simulink model "Black_box_system_2_1_3"  (R2025b)
settings: Solver=VariableStepAuto  StartTime=0.0  StopTime=20  FixedStep=0.001  RelTol=1e-3
undefined symbols (not defined in the file): Beq, degs2rpm, drv, gbox, Jeq, K_W, kd, ki, kp, mld, mot, rdp, Req, sens, tl, u_bar_max
libraries: simulink x1
settings Model: Creator=Enrico  LastModifiedBy=Enrico
settings DataIOCC: ReturnWorkspaceOutputsName=out_black_box

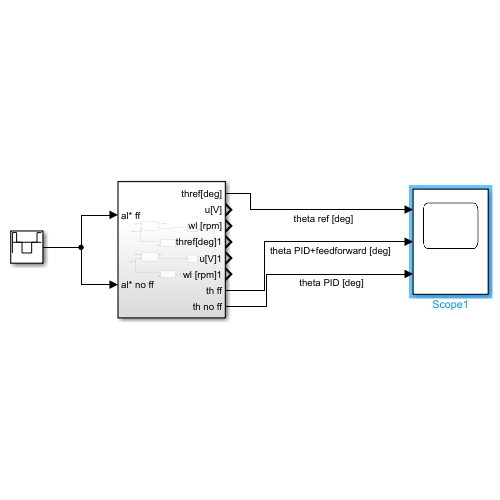
[thumbnail: Simulink's stored preview of the top-level diagram]
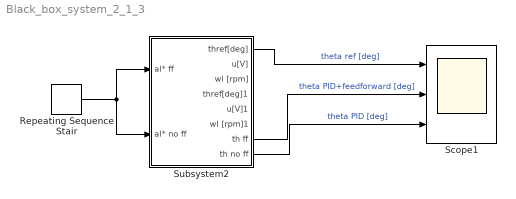
== system Black_box_system_2_1_3 ==
  Repeating Sequence Stair : simulink/Sources/Repeating Sequence Stair  OutValues=[900 0 -900 -900 0 900]  tsamp=0.5  OutMin=[]  OutMax=[]  OutDataTypeStr=double  OutputDataTypeScalingMode=double  OutDataType=fixdt(0,8)  ConRadixGroup=Best Precision: Vector-wise  OutScaling=2^-12
  Scope1 : Scope  NumInputPorts=3
      settings: ActiveDisplayYMinimum=2541.6022792553317  ActiveDisplayYMaximum=2555.3739505789249
  Subsystem2 : Subsystem
  wires:
  Repeating Sequence Stair/1 -> Subsystem2/2(al* no ff), Subsystem2/1(al* ff)
  Subsystem2/1(thref[deg]) -> Scope1/1  "theta ref [deg]"
  Subsystem2/8(th no ff) -> Scope1/3  "theta PID [deg]"
  Subsystem2/7(th ff) -> Scope1/2  "theta PID+feedforward [deg]"

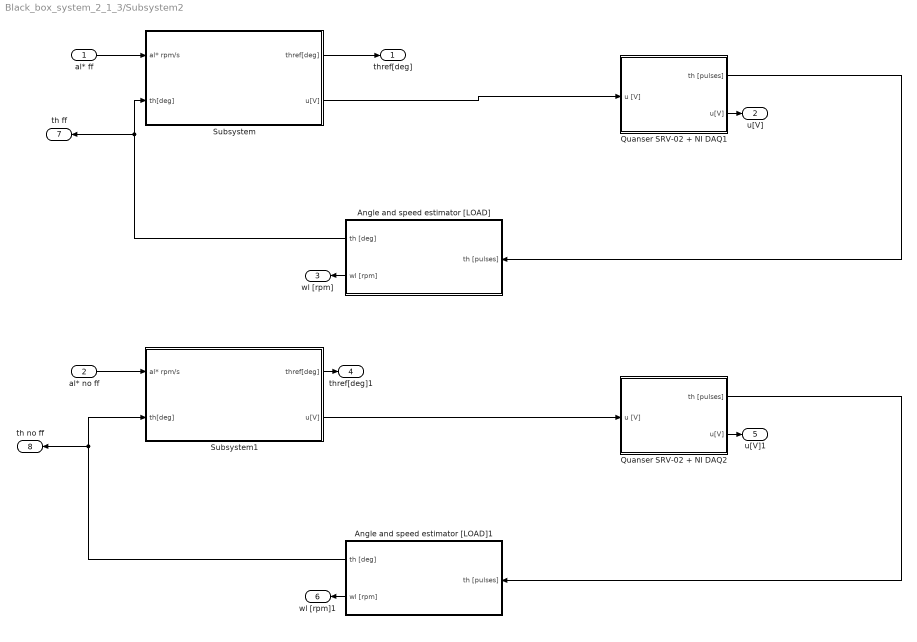
== system Black_box_system_2_1_3/Subsystem2 ==
  al* ff : Inport
  al* no ff : Inport  Port=2
  Angle and speed estimator [LOAD] : Subsystem
  Angle and speed estimator [LOAD]1 : Subsystem
  Quanser SRV-02 + NI DAQ1 : Subsystem  mask(Quanser SRV-02 (with inertial load) + NI DAQ){Ts=0.001, fricType=Karnopp}
      mask prompts: Ts "NI DAQ Sample Time:"; fricType "Friction model"
      mask help: Quanser SRV-02 (with inertial load) + NI DAQ model.
      mask init:
      | %%  Sensors data
      | 
      | %   shunt resistor
      | sens.curr.Rs = 0.5;                         %   resistance [Ohm]   
      | sens.curr.uRs_std = 0.01;                   %   voltage noise standard dev [V]                           
      | sens.curr.uRs_var = sens.curr.uRs_std^2;	%   voltage noise variance [V^2]
      | 
      | %   Hewlett-Packard HEDS-5540#A06 optical encoder
      | sens.enc.ppr = 500*4;                       %   pulses per rotation
      | sens.enc.pulse2deg = 360/sens.enc.ppr;      %   [pulses] -> [deg]
      | sens.enc.pulse2rad = 2*pi/sens.enc.ppr;     %   [pulses] -> [rad]
      | sens.enc.deg2pulse = sens.enc.ppr/360;      %   [deg] -> [pulses]
      | sens.enc.rad2pulse = sens.enc.ppr/2/pi;     %   [rad] -> [pulses]
      | 
      | 
      | %%  Data acquisition board (daq) data
      | 
      | %   NI PCI-6221 DAC data
      | daq.dac.bits = 16;                                  %   resolution (bits)
      | daq.dac.fs   = 10;                                  %   full scale 
      | daq.dac.q    = 2*daq.dac.fs/(2^daq.dac.bits-1);     %	quantization
      | 
      | %   NI PCI-6221 ADC data
      | daq.adc.bits = 16;                                  %   resolution (bits)
      | daq.adc.fs   = 10;                                  %   full scale (as set in SLDRT Analog Input block)
      | daq.adc.q    = 2*daq.adc.fs/(2^daq.adc.bits-1);     %   quantization
      mask Help:
      | Riccardo Antonello (antonello@dei.unipd.it)
      | 
      | April 24, 2020
      | 
      | Dept. of Information Engineering, University of Padova
      mask TypeOptions fricType: Coulomb + viscous | Karnopp
  Quanser SRV-02 + NI DAQ2 : Subsystem  mask(Quanser SRV-02 (with inertial load) + NI DAQ){Ts=0.001, fricType=Karnopp}
      mask prompts: Ts "NI DAQ Sample Time:"; fricType "Friction model"
      mask help: Quanser SRV-02 (with inertial load) + NI DAQ model.
      mask init: same as Black_box_system_2_1_3/Subsystem2/Quanser SRV-02 + NI DAQ1
      mask Help:
      | Riccardo Antonello (antonello@dei.unipd.it)
      | 
      | April 24, 2020
      | 
      | Dept. of Information Engineering, University of Padova
      mask TypeOptions fricType: Coulomb + viscous | Karnopp
  Subsystem : Subsystem
  Subsystem1 : Subsystem
  thref[deg] : Outport
  u[V] : Outport  Port=2
  wl [rpm] : Outport  Port=3
  thref[deg]1 : Outport  Port=4
  u[V]1 : Outport  Port=5
  wl [rpm]1 : Outport  Port=6
  th ff : Outport  Port=7
  th no ff : Outport  Port=8
  wires:
  Subsystem/2(u[V]) -> Quanser SRV-02 + NI DAQ1/1(u [V])
  al* no ff/1 -> Subsystem1/1(al* rpm/s)
  Quanser SRV-02 + NI DAQ1/1(th [pulses]) -> Angle and speed estimator [LOAD]/1(th [pulses])
  Angle and speed estimator [LOAD]1/1(th [deg]) -> Subsystem1/2(th[deg]), th no ff/1
  Subsystem1/2(u[V]) -> Quanser SRV-02 + NI DAQ2/1(u [V])
  Quanser SRV-02 + NI DAQ2/2(u[V]) -> u[V]1/1
  Quanser SRV-02 + NI DAQ2/1(th [pulses]) -> Angle and speed estimator [LOAD]1/1(th [pulses])
  Angle and speed estimator [LOAD]/1(th [deg]) -> th ff/1, Subsystem/2(th[deg])
  Subsystem/1(thref[deg]) -> thref[deg]/1
  al* ff/1 -> Subsystem/1(al* rpm/s)
  Angle and speed estimator [LOAD]1/2(wl [rpm]) -> wl [rpm]1/1
  Angle and speed estimator [LOAD]/2(wl [rpm]) -> wl [rpm]/1
  Subsystem1/1(thref[deg]) -> thref[deg]1/1
  Quanser SRV-02 + NI DAQ1/2(u[V]) -> u[V]/1

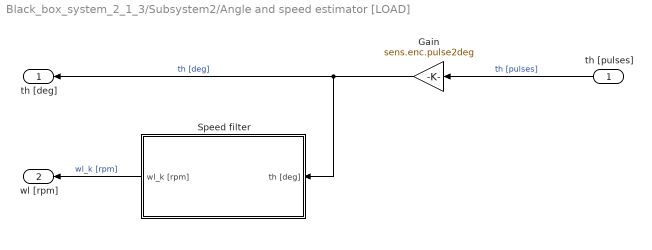
== system Black_box_system_2_1_3/Subsystem2/Angle and speed estimator [LOAD] ==
  th [pulses] : Inport
  Gain : Gain  Gain=sens.enc.pulse2deg
  Speed filter : Subsystem
  th [deg] : Outport
  wl [rpm] : Outport  Port=2
  wires:
  Speed filter/1(wl_k [rpm]) -> wl [rpm]/1  "wl_k [rpm]"
  th [pulses]/1 -> Gain/1  "th [pulses]"
  Gain/1 -> Speed filter/1(th [deg]), th [deg]/1  "th [deg]"

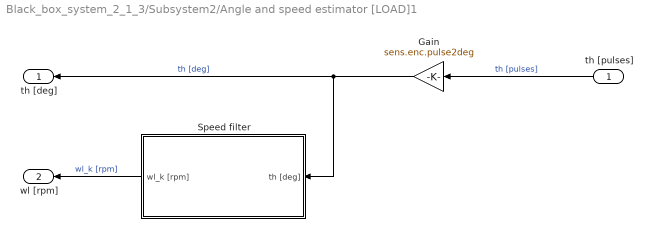
== system Black_box_system_2_1_3/Subsystem2/Angle and speed estimator [LOAD]1 ==
  th [pulses] : Inport
  Gain : Gain  Gain=sens.enc.pulse2deg
  Speed filter : Subsystem
  th [deg] : Outport
  wl [rpm] : Outport  Port=2
  wires:
  Speed filter/1(wl_k [rpm]) -> wl [rpm]/1  "wl_k [rpm]"
  th [pulses]/1 -> Gain/1  "th [pulses]"
  Gain/1 -> Speed filter/1(th [deg]), th [deg]/1  "th [deg]"

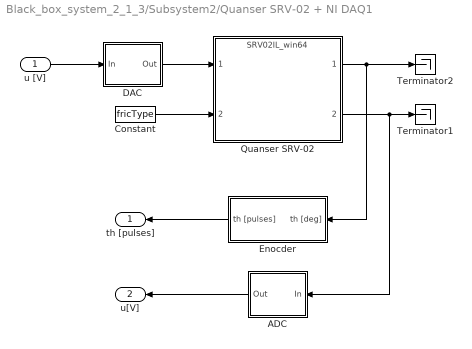
== system Black_box_system_2_1_3/Subsystem2/Quanser SRV-02 + NI DAQ1 ==
  u [V] : Inport
  ADC : Subsystem
  Constant : Constant  Value=fricType
  DAC : Subsystem
  Enocder : Subsystem
  Quanser SRV-02 : ModelReference  ModelNameDialog=SRV02IL_win64.slxp  ModelReferenceVersion=1.44  CopyOfModelProtected=on
  Terminator1 : Terminator
  Terminator2 : Terminator
  th [pulses] : Outport
  u[V] : Outport  Port=2
  wires:
  Enocder/1(th [pulses]) -> th [pulses]/1
  ADC/1(Out) -> u[V]/1
  DAC/1(Out) -> Quanser SRV-02/1
  Quanser SRV-02/2 -> ADC/1(In), Terminator1/1
  u [V]/1 -> DAC/1(In)
  Quanser SRV-02/1 -> Enocder/1(th [deg]), Terminator2/1
  Constant/1 -> Quanser SRV-02/2

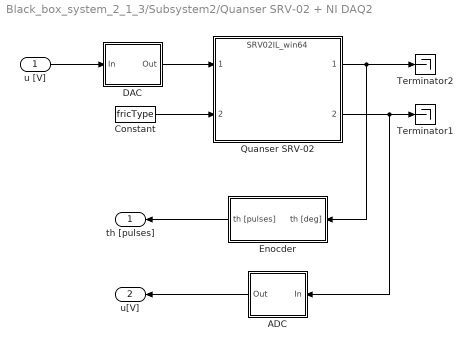
== system Black_box_system_2_1_3/Subsystem2/Quanser SRV-02 + NI DAQ2 ==
  u [V] : Inport
  ADC : Subsystem
  Constant : Constant  Value=fricType
  DAC : Subsystem
  Enocder : Subsystem
  Quanser SRV-02 : ModelReference  ModelNameDialog=SRV02IL_win64.slxp  ModelReferenceVersion=1.44  CopyOfModelProtected=on
  Terminator1 : Terminator
  Terminator2 : Terminator
  th [pulses] : Outport
  u[V] : Outport  Port=2
  wires:
  Enocder/1(th [pulses]) -> th [pulses]/1
  ADC/1(Out) -> u[V]/1
  DAC/1(Out) -> Quanser SRV-02/1
  Quanser SRV-02/2 -> ADC/1(In), Terminator1/1
  u [V]/1 -> DAC/1(In)
  Quanser SRV-02/1 -> Enocder/1(th [deg]), Terminator2/1
  Constant/1 -> Quanser SRV-02/2

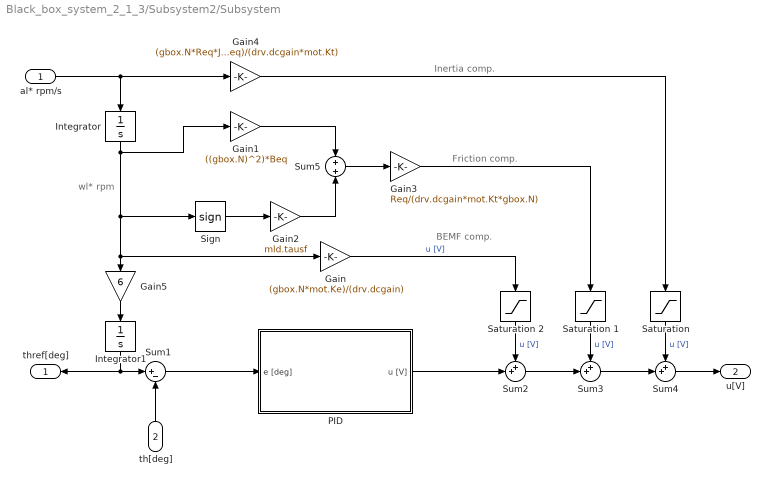
== system Black_box_system_2_1_3/Subsystem2/Subsystem ==
  note: rpm
  note: Inertia comp.
  note: Friction comp.
  note: BEMF comp.
  note: wl*
  al* rpm/s : Inport
  th[deg] : Inport  Port=2
  Gain : Gain  Gain=(gbox.N*mot.Ke)/(drv.dcgain)
  Gain1 : Gain  Gain=((gbox.N)^2)*Beq
  Gain2 : Gain  Gain=mld.tausf
  Gain3 : Gain  Gain=Req/(drv.dcgain*mot.Kt*gbox.N)
  Gain4 : Gain  Gain=(gbox.N*Req*Jeq)/(drv.dcgain*mot.Kt)
  Gain5 : Gain  Gain=6
  Integrator : Integrator
  Integrator1 : Integrator
  PID : Subsystem
  "Saturation " : Saturate  UpperLimit=u_bar_max  LowerLimit=-u_bar_max
  Saturation 1 : Saturate  UpperLimit=u_bar_max  LowerLimit=-u_bar_max
  Saturation 2 : Saturate  UpperLimit=u_bar_max  LowerLimit=-u_bar_max
  Sign : Signum
  Sum1 : Sum  Inputs=|+-
  Sum2 : Sum  Inputs=++|
  Sum3 : Sum  Inputs=++|
  Sum4 : Sum  Inputs=++|
  Sum5 : Sum  Inputs=+|+
  thref[deg] : Outport
  u[V] : Outport  Port=2
  wires:
  Sum3/1 -> Sum4/2
  Gain2/1 -> Sum5/2
  Integrator/1 -> Sign/1, Gain5/1, Gain/1, Gain1/1
  Sum2/1 -> Sum3/2
  Sum4/1 -> u[V]/1
  Integrator1/1 -> thref[deg]/1, Sum1/1
  Saturation 1/1 -> Sum3/1  "u [V]"
  PID/1(u [V]) -> Sum2/2
  Sum5/1 -> Gain3/1
  Gain1/1 -> Sum5/1
  Gain5/1 -> Integrator1/1
  Sign/1 -> Gain2/1
  Saturation 2/1 -> Sum2/1  "u [V]"
  Sum1/1 -> PID/1(e [deg])
  "Saturation "/1 -> Sum4/1  "u [V]"
  al* rpm/s/1 -> Gain4/1, Integrator/1
  th[deg]/1 -> Sum1/2
  Gain4/1 -> "Saturation "/1
  Gain3/1 -> Saturation 1/1
  Gain/1 -> Saturation 2/1  "u [V]"

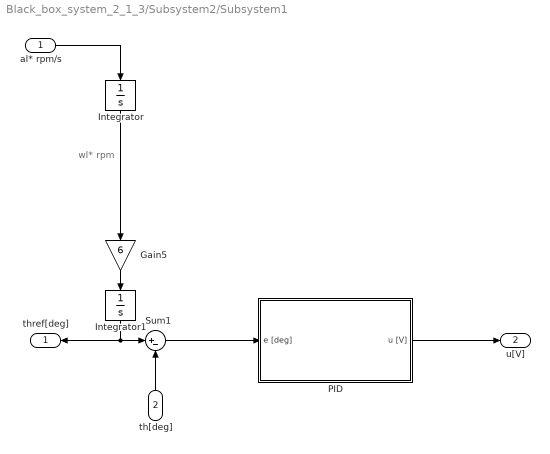
== system Black_box_system_2_1_3/Subsystem2/Subsystem1 ==
  note: rpm
  note: wl*
  al* rpm/s : Inport
  th[deg] : Inport  Port=2
  Gain5 : Gain  Gain=6
  Integrator : Integrator
  Integrator1 : Integrator
  PID : Subsystem
  Sum1 : Sum  Inputs=|+-
  thref[deg] : Outport
  u[V] : Outport  Port=2
  wires:
  Integrator/1 -> Gain5/1
  Integrator1/1 -> thref[deg]/1, Sum1/1
  Gain5/1 -> Integrator1/1
  Sum1/1 -> PID/1(e [deg])
  al* rpm/s/1 -> Integrator/1
  th[deg]/1 -> Sum1/2
  PID/1(u [V]) -> u[V]/1

== system Black_box_system_2_1_3/Subsystem2/Angle and speed estimator [LOAD]/Speed filter ==
  th [deg] : Inport
  Real Derivative : TransferFcn  Numerator=[rdp.wci^2 0]  Denominator=[1 2*rdp.di*rdp.wci rdp.wci^2]
  degs2rpm : Gain  Gain=degs2rpm
  wl_k [rpm] : Outport
  wires:
  th [deg]/1 -> Real Derivative/1
  degs2rpm/1 -> wl_k [rpm]/1  "wl-meas"
  Real Derivative/1 -> degs2rpm/1

== system Black_box_system_2_1_3/Subsystem2/Angle and speed estimator [LOAD]1/Speed filter ==
  th [deg] : Inport
  Real Derivative : TransferFcn  Numerator=[rdp.wci^2 0]  Denominator=[1 2*rdp.di*rdp.wci rdp.wci^2]
  degs2rpm : Gain  Gain=degs2rpm
  wl_k [rpm] : Outport
  wires:
  th [deg]/1 -> Real Derivative/1
  degs2rpm/1 -> wl_k [rpm]/1  "wl-meas"
  Real Derivative/1 -> degs2rpm/1

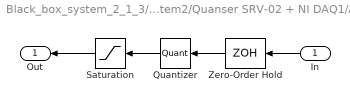
== system Black_box_system_2_1_3/Subsystem2/Quanser SRV-02 + NI DAQ1/ADC ==
  In : Inport
  Quantizer : Quantizer  QuantizationInterval=daq.adc.q
  Saturation : Saturate  UpperLimit=daq.adc.fs  LowerLimit=-daq.adc.fs
  Zero-Order Hold : ZeroOrderHold  SampleTime=Ts
  Out : Outport
  wires:
  Saturation/1 -> Out/1
  In/1 -> Zero-Order Hold/1
  Quantizer/1 -> Saturation/1
  Zero-Order Hold/1 -> Quantizer/1

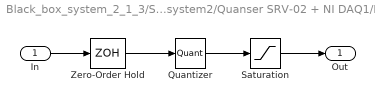
== system Black_box_system_2_1_3/Subsystem2/Quanser SRV-02 + NI DAQ1/DAC ==
  In : Inport
  Quantizer : Quantizer  QuantizationInterval=daq.dac.q
  Saturation : Saturate  UpperLimit=daq.dac.fs  LowerLimit=-daq.dac.fs
  Zero-Order Hold : ZeroOrderHold  SampleTime=Ts
  Out : Outport
  wires:
  Quantizer/1 -> Saturation/1
  In/1 -> Zero-Order Hold/1
  Zero-Order Hold/1 -> Quantizer/1
  Saturation/1 -> Out/1

== system Black_box_system_2_1_3/Subsystem2/Quanser SRV-02 + NI DAQ1/Enocder ==
  th [deg] : Inport
  Quantizer : Quantizer  QuantizationInterval=sens.enc.pulse2deg
  Zero-Order Hold : ZeroOrderHold  SampleTime=Ts
  deg2pulse : Gain  Gain=sens.enc.deg2pulse
  th [pulses] : Outport
  wires:
  Quantizer/1 -> deg2pulse/1
  th [deg]/1 -> Zero-Order Hold/1
  Zero-Order Hold/1 -> Quantizer/1
  deg2pulse/1 -> th [pulses]/1

== system Black_box_system_2_1_3/Subsystem2/Quanser SRV-02 + NI DAQ2/ADC ==
  In : Inport
  Quantizer : Quantizer  QuantizationInterval=daq.adc.q
  Saturation : Saturate  UpperLimit=daq.adc.fs  LowerLimit=-daq.adc.fs
  Zero-Order Hold : ZeroOrderHold  SampleTime=Ts
  Out : Outport
  wires:
  Saturation/1 -> Out/1
  In/1 -> Zero-Order Hold/1
  Quantizer/1 -> Saturation/1
  Zero-Order Hold/1 -> Quantizer/1

== system Black_box_system_2_1_3/Subsystem2/Quanser SRV-02 + NI DAQ2/DAC ==
  In : Inport
  Quantizer : Quantizer  QuantizationInterval=daq.dac.q
  Saturation : Saturate  UpperLimit=daq.dac.fs  LowerLimit=-daq.dac.fs
  Zero-Order Hold : ZeroOrderHold  SampleTime=Ts
  Out : Outport
  wires:
  Quantizer/1 -> Saturation/1
  In/1 -> Zero-Order Hold/1
  Zero-Order Hold/1 -> Quantizer/1
  Saturation/1 -> Out/1

== system Black_box_system_2_1_3/Subsystem2/Quanser SRV-02 + NI DAQ2/Enocder ==
  th [deg] : Inport
  Quantizer : Quantizer  QuantizationInterval=sens.enc.pulse2deg
  Zero-Order Hold : ZeroOrderHold  SampleTime=Ts
  deg2pulse : Gain  Gain=sens.enc.deg2pulse
  th [pulses] : Outport
  wires:
  Quantizer/1 -> deg2pulse/1
  th [deg]/1 -> Zero-Order Hold/1
  Zero-Order Hold/1 -> Quantizer/1
  deg2pulse/1 -> th [pulses]/1

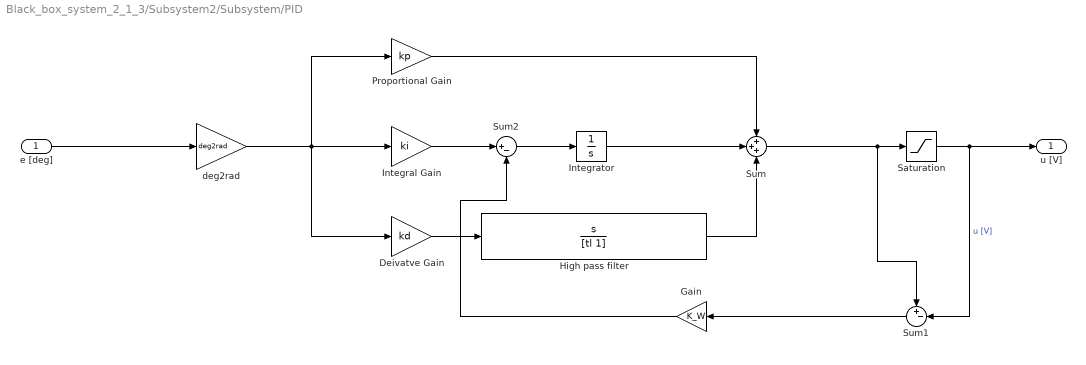
== system Black_box_system_2_1_3/Subsystem2/Subsystem/PID ==
  e [deg] : Inport
  Deivatve Gain : Gain  Gain=kd
  Gain : Gain  Gain=K_W
  High pass filter : TransferFcn  Numerator=[1 0]  Denominator=[tl 1]
  Integral Gain : Gain  Gain=ki
  Integrator : Integrator
  Proportional Gain : Gain  Gain=kp
  "Saturation " : Saturate  UpperLimit=u_bar_max  LowerLimit=-u_bar_max
  Sum : Sum  Inputs=+++
  Sum1 : Sum  Inputs=+-|
  Sum2 : Sum  Inputs=|+-
  deg2rad : Gain  Gain=deg2rad
  u [V] : Outport
  wires:
  Deivatve Gain/1 -> High pass filter/1
  e [deg]/1 -> deg2rad/1
  Integrator/1 -> Sum/2
  "Saturation "/1 -> Sum1/2, u [V]/1  "u [V]"
  deg2rad/1 -> Deivatve Gain/1, Proportional Gain/1, Integral Gain/1
  High pass filter/1 -> Sum/3
  Proportional Gain/1 -> Sum/1
  Sum/1 -> Sum1/1, "Saturation "/1
  Sum1/1 -> Gain/1
  Integral Gain/1 -> Sum2/1
  Sum2/1 -> Integrator/1
  Gain/1 -> Sum2/2

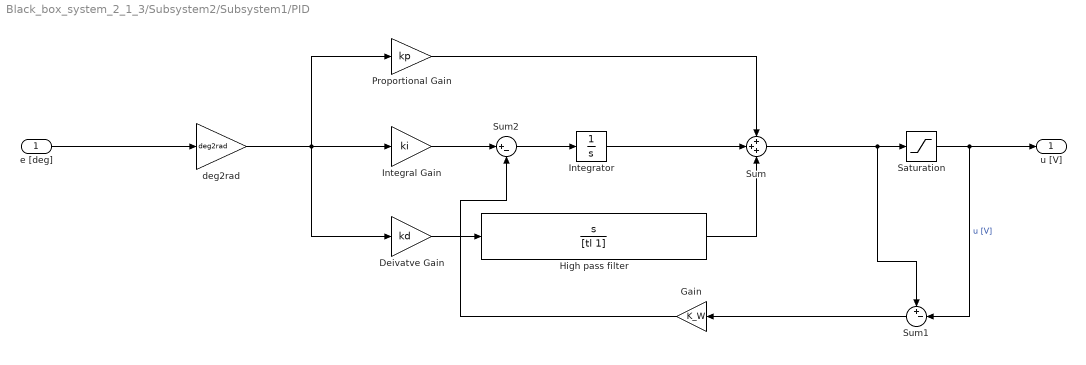
== system Black_box_system_2_1_3/Subsystem2/Subsystem1/PID ==
  e [deg] : Inport
  Deivatve Gain : Gain  Gain=kd
  Gain : Gain  Gain=K_W
  High pass filter : TransferFcn  Numerator=[1 0]  Denominator=[tl 1]
  Integral Gain : Gain  Gain=ki
  Integrator : Integrator
  Proportional Gain : Gain  Gain=kp
  "Saturation " : Saturate  UpperLimit=u_bar_max  LowerLimit=-u_bar_max
  Sum : Sum  Inputs=+++
  Sum1 : Sum  Inputs=+-|
  Sum2 : Sum  Inputs=|+-
  deg2rad : Gain  Gain=deg2rad
  u [V] : Outport
  wires:
  Deivatve Gain/1 -> High pass filter/1
  e [deg]/1 -> deg2rad/1
  Integrator/1 -> Sum/2
  "Saturation "/1 -> Sum1/2, u [V]/1  "u [V]"
  deg2rad/1 -> Deivatve Gain/1, Proportional Gain/1, Integral Gain/1
  High pass filter/1 -> Sum/3
  Proportional Gain/1 -> Sum/1
  Sum/1 -> Sum1/1, "Saturation "/1
  Sum1/1 -> Gain/1
  Integral Gain/1 -> Sum2/1
  Sum2/1 -> Integrator/1
  Gain/1 -> Sum2/2
